simulink model "myModel"  (R2023b)
settings: Solver=VariableStepAuto  StartTime=0.0  StopTime=10.0  RelTol=1e-3
settings Model: Creator=Jose  LastModifiedBy=Jose

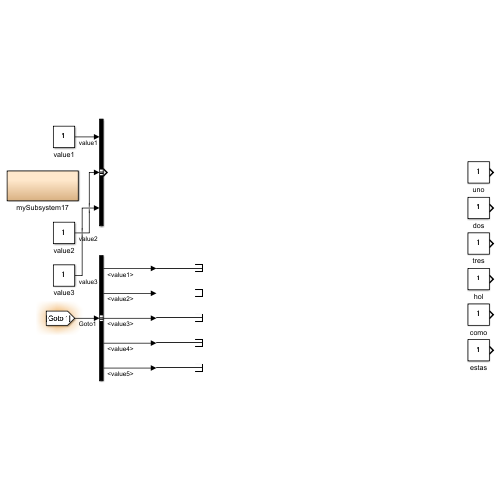
[thumbnail: Simulink's stored preview of the top-level diagram]
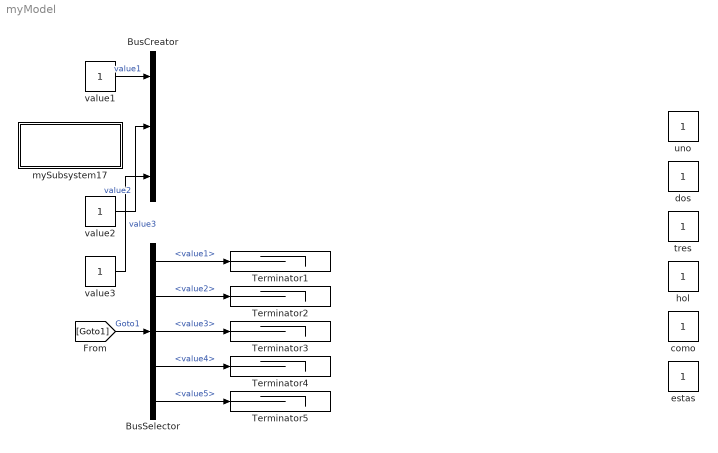
== system myModel ==
  BusCreator : BusCreator  Inputs=3
  BusSelector : BusSelector  OutputSignals=value1,value2,value3,value4,value5
  Terminator{1..5} (5 alike) : Terminator
  como : Constant
  dos : Constant
  estas : Constant
  hol : Constant
  mySubsystem17 : Subsystem
  tres : Constant
  uno : Constant
  value1 : Constant
  value2 : Constant
  value3 : Constant
  wires:
  BusSelector/2 -> Terminator2/1  "<value2>"
  value1/1 -> BusCreator/1  "value1"
  value3/1 -> BusCreator/3  "value3"
  value2/1 -> BusCreator/2  "value2"
  BusSelector/4 -> Terminator4/1  "<value4>"
  [Goto1] -> BusSelector/1  "Goto1"
  BusSelector/1 -> Terminator1/1  "<value1>"
  BusSelector/3 -> Terminator3/1  "<value3>"
  BusSelector/5 -> Terminator5/1  "<value5>"

== system myModel/mySubsystem17 ==
